simulink model "mbed_flash_constants"  (R2015a)
settings: Solver=FixedStepDiscrete  SolverMode=SingleTasking  StartTime=0.0  StopTime=10.0  FixedStep=1e-3  RelTol=1e-3
values from neighbouring files (symbols this model uses):
  Param1 = 1.0    [mbed_flash_constants.sldd]
libraries: mbed_targets_stm_disco_f429 x2, simulink x1
settings Model: DataDictionary=mbed_flash_constants.sldd  Creator=oh  LastModifiedBy=oh
settings OptimizationCC: InlineParams=on  OptimizeModelRefInitCode=on  LifeSpan=1
settings HardwareCC: ProdLargestAtomicInteger=Long  ProdLargestAtomicFloat=Double  ProdEndianess=LittleEndian  ProdHWDeviceType=ARM Compatible->ARM Cortex
settings RTWCC: SystemTargetFile=mbed.tlc  GenCodeOnly=on  TemplateMakefile=mbed.tmf  Description=Mbed Target (Embedded Target)  TargetLang=C++
settings CodeAppCC: IgnoreCustomStorageClasses=off
settings STFCustomTargetCC: CombineOutputUpdateFcns=on  SupportVariableSizeSignals=off  SystemTargetFile=mbed.tlc
settings ERTTargetCC: SupportVariableSizeSignals=off  ERTCustomFileTemplate=mbed_file_process.tlc  MemSecPackage=Simulink  MemSecDataConstants=MemConst  MemSecDataParameters=MemConst

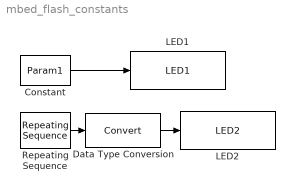
== system mbed_flash_constants ==
  Constant : Constant  Value=Param1
  Data Type Conversion : DataTypeConversion
  LED1 : mbed_targets_stm_disco_f429/LED1  Parameter1=0
  LED2 : mbed_targets_stm_disco_f429/LED2  Parameter1=0
  Repeating Sequence : simulink/Sources/Repeating Sequence  rep_seq_t=Param2  rep_seq_y=Param3
  wires:
  Constant/1 -> LED1/1
  Repeating Sequence/1 -> Data Type Conversion/1
  Data Type Conversion/1 -> LED2/1
